simulink model "SWC_FDC_type"  (R2021b)
settings: Solver=FixedStepDiscrete  StartTime=0.0  StopTime=10.0  FixedStep=0.001  RelTol=1e-3
values from neighbouring files (symbols this model uses):
  DID_VCUKey = uint16(0x0202)    [vcu_local_hdr.m]
  DID_XWD = uint16(513)    [vcu_local_hdr.m]
  DIDLen_DKCKey = uint16(8)    [vcu_local_hdr.m]
  DIDLen_DynoMode = uint16(1)    [vcu_local_hdr.m]
  DIDLen_LFLowPresThre = uint16(1)    [vcu_local_hdr.m]
  DIDLen_LFSensorID = uint16(4)    [vcu_local_hdr.m]
  DIDLen_LRLowPresThre = uint16(1)    [vcu_local_hdr.m]
  DIDLen_LRSensorID = uint16(4)    [vcu_local_hdr.m]
  DIDLen_RFLowPresThre = uint16(1)    [vcu_local_hdr.m]
  DIDLen_RFSensorID = uint16(4)    [vcu_local_hdr.m]
  DIDLen_RRLowPresThre = uint16(1)    [vcu_local_hdr.m]
  DIDLen_RRSensorID = uint16(4)    [vcu_local_hdr.m]
  DIDLen_SensorMode = uint16(1)    [vcu_local_hdr.m]
  DIDLen_TPMSLearnSta = uint16(1)    [vcu_local_hdr.m]
  DIDLen_WhlPres = uint16(4)    [vcu_local_hdr.m]
  DIDLen_WhlSensorBattSta = uint16(1)    [vcu_local_hdr.m]
  DIDLen_WhlTmp = uint16(4)    [vcu_local_hdr.m]
  DIDLen_XWDMode = uint16(1)    [vcu_local_hdr.m]
  DIDNum_DKCKey = uint16(0x0202)    [vcu_local_hdr.m]
  DIDNum_DynoMode = uint16(0x0203)    [vcu_local_hdr.m]
  DIDNum_LFLowPresThre = uint16(0x0B08)    [vcu_local_hdr.m]
  DIDNum_LFSensorID = uint16(0x0B01)    [vcu_local_hdr.m]
  DIDNum_LRLowPresThre = uint16(0x0B0A)    [vcu_local_hdr.m]
  DIDNum_LRSensorID = uint16(0x0B03)    [vcu_local_hdr.m]
  DIDNum_RFLowPresThre = uint16(0x0B09)    [vcu_local_hdr.m]
  DIDNum_RFSensorID = uint16(0x0B02)    [vcu_local_hdr.m]
  DIDNum_RRLowPresThre = uint16(0x0B0B)    [vcu_local_hdr.m]
  DIDNum_RRSensorID = uint16(0x0B04)    [vcu_local_hdr.m]
  DIDNum_SensorMode = uint16(0x0B0C)    [vcu_local_hdr.m]
  DIDNum_TPMSLearnSta = uint16(0x0B0D)    [vcu_local_hdr.m]
  DIDNum_WhlPres = uint16(0x0B05)    [vcu_local_hdr.m]
  DIDNum_WhlSensorBattSta = uint16(0x0B07)    [vcu_local_hdr.m]
  DIDNum_WhlTmp = uint16(0x0B06)    [vcu_local_hdr.m]
  DIDNum_XWDMode = uint16(0x0201)    [vcu_local_hdr.m]
  DIDVCUKeyLength = uint16(8)    [vcu_local_hdr.m]
  ENUM_DRIVETRAIN_AWD = uint8(  2  )    [vcu_local_hdr.m]
  ENUM_DRIVETRAIN_FWD = uint8(  1  )    [vcu_local_hdr.m]
  ENUM_DRIVETRAIN_RWD = uint8(  0  )    [vcu_local_hdr.m]
  ENUM_TPMSLearnStatus_LEARNED = uint8(  1  )    [vcu_local_hdr.m]
  ENUM_TPMSLearnStatus_LEARNFAIL = uint8(  2  )    [vcu_local_hdr.m]
  ENUM_TPMSLearnStatus_NOTLEARN = uint8(  0  )    [vcu_local_hdr.m]
  ENUM_TPMSSTA_FAT = uint8(  8  )    [vcu_local_hdr.m]
  ENUM_TPMSSTA_LOWBATTERY = uint8(  2  )    [vcu_local_hdr.m]
  FALSE = boolean( 0 )    [vcu_local_hdr.m]
  ONE_INT = uint8(1)    [vcu_local_hdr.m]
  P_boolean = 0.0    [APPTypes.sldd]
  TRUE = boolean( 1 )    [vcu_local_hdr.m]
  ZERO_FLOAT = single(0)    [vcu_local_hdr.m]
  ZERO_INT = uint8(0)    [vcu_local_hdr.m]
undefined symbols (not defined in the file or in its folder): f32_ApsOutVehSpdSig, KHAL_DKCDecryptEnable_flg_ovrdflg, KHAL_DKCDecryptEnable_flg_ovrdval, KHAL_RandomNumberY1_enum, KHAL_RandomNumberY2_enum, KHAL_RandomNumberY_ovrdflg, KHAL_TPMSRESBUTT_flg_ovrdflg, KHAL_TPMSRESBUTT_flg_ovrdval, R_DIDWriteCDD_CSOP_DIDSet_DKCKey, R_DIDWriteCDD_CSOP_DIDSet_DynoMode, R_DIDWriteCDD_CSOP_DIDSet_LFLowPresThre, R_DIDWriteCDD_CSOP_DIDSet_LFSensorID, R_DIDWriteCDD_CSOP_DIDSet_LRLowPresThre, R_DIDWriteCDD_CSOP_DIDSet_LRSensorID, R_DIDWriteCDD_CSOP_DIDSet_RFLowPresThre, R_DIDWriteCDD_CSOP_DIDSet_RFSensorID, R_DIDWriteCDD_CSOP_DIDSet_RRLowPresThre, R_DIDWriteCDD_CSOP_DIDSet_RRSensorID, R_DIDWriteCDD_CSOP_DIDSet_SensorMode, R_DIDWriteCDD_CSOP_DIDSet_TPMSLearnSta, R_DIDWriteCDD_CSOP_DIDSet_WhlPres, R_DIDWriteCDD_CSOP_DIDSet_WhlSensorBattSta, R_DIDWriteCDD_CSOP_DIDSet_WhlTmp, R_DIDWriteCDD_CSOP_DIDSet_XWDMode, R_E2E_CAN3_VCU1_CSOP_Write_CAN3_VCU1, R_E2E_CAN4_VCU1_CSOP_Write_CAN4_VCU1, R_FDCCDD_Inner_CSOP_FDC_AppCallSleep, R_HALIN_IMU_CSOP_IMUSetSta, R_HALINCDD_CSOP_PAS_Handler, R_HALINCDD_CSOP_UDS_Main, R_HALOUT_APS_CSOP_ApsOutput, R_HALOUTCDD_CSOP_AppNmStateReq, R_HALOUTCDD_CSOP_IVIReset, R_HALOUTCDD_CSOP_SetAcoreRebootCmdACK, R_HALOUTCDD_CSOP_SetSysPwrStat, R_HALOUTCDD_CSOP_SleepRequest, R_NVMReadCDD_Inner_NVM_ReadOperation, R_NVMWriteCDD_Inner_NVM_WriteOperation, R_UDSCDD_CSOP_DdmRestartOperationCycle, R_WDGCDD_CSOP_Call_Watchdog, R_WDGCDD_CSOP_Call_WDG_AppEnd, R_WDGCDD_CSOP_Call_WDG_AppStart, u16_DIDLen_DKCKey, u16_DIDLen_DynoMode, u16_DIDLen_LFLowPresThre, u16_DIDLen_LFSensorID, u16_DIDLen_LRLowPresThre, u16_DIDLen_LRSensorID, u16_DIDLen_RFLowPresThre, u16_DIDLen_RFSensorID, u16_DIDLen_RRLowPresThre, u16_DIDLen_RRSensorID, u16_DIDLen_SensorMode, u16_DIDLen_TPMSLearnSta, u16_DIDLen_WhlPres, u16_DIDLen_WhlSensorBattSta, u16_DIDLen_WhlTmp, u16_DIDLen_XWDMode, u16_DIDNum_DKCKey, u16_DIDNum_DynoMode ... (+42)
libraries: simulink x215, FVT_lib x137, hcu_lib x12, hdlsllib x9, app x1, halin x1, halout x1, inp x1, outp x1
(part 1 of 11)
settings Model: DataDictionary=APPTypes.sldd  Creator=FVT23118  LastModifiedBy=FVT23118
settings DataIOCC: SaveFormat=StructureWithTime
settings OptimizationCC: DefaultParameterBehavior=Inlined  EnhancedBackFolding=on  PassReuseOutputArgsAs=Individual arguments  ZeroExternalMemoryAtStartup=off  ZeroInternalMemoryAtStartup=off  OptimizeBlockOrder=speed  DifferentSizesBufferReuse=on  OptimizationCustomize=off  EfficientTunableParamExpr=on
settings DebuggingCC: ParameterTunabilityLossMsg=error
settings HardwareCC: ProdBitPerPointer=32  ProdBitPerSizeT=32  ProdBitPerPtrDiffT=32  ProdLargestAtomicInteger=Long  ProdLargestAtomicFloat=Double  ProdWordSize=32  ProdLongLongMode=on  ProdHWDeviceType=ARM Compatible->ARM Cortex-M
settings ModelReferenceCC: ModelReferenceNumInstancesAllowed=Single
settings SFSimCC: MATLABDynamicMemAlloc=off
settings RTWCC: Description=AUTOSAR  SystemTargetFile=autosar.tlc  GenCodeOnly=on  TemplateMakefile=ert_default_tmf  PortableWordSizes=on
settings CodeAppCC: ForceParamTrailComments=on  IgnoreCustomStorageClasses=off  OperatorAnnotations=on  SimulinkDataObjDesc=on  SFDataObjDesc=on  InsertBlockDesc=on
settings STFCustomTargetCC: TargetLangStandard=C99 (ISO)  MultiwordLength=256  ParMdlRefBuildCompliant=on  CompOptLevelCompliant=on  IncludeMdlTerminateFcn=off  CombineOutputUpdateFcns=on  SuppressErrorStatus=on  ERTCustomFileBanners=on  SupportNonFinite=off  SupportComplex=off  SupportContinuousTime=off  SupportNonInlinedSFcns=off  RemoveResetFunc=on  MATLABClassNameForMDSCustomization=Simulink.SoftwareTarget.ERTCustomization  AutosarCompliant=on  GRTInterface=off  UseToolchainInfoCompliant=on  LookupTableObjectStructAxisOrder=2,1,3,4,...  LUTObjectStructOrderEvenSpacing=Size,Table,Breakpoints  SystemTargetFile=autosar.tlc
settings ERTTargetCC: TargetLangStandard=C99 (ISO)  ConcurrentExecutionCompliant=off  IncludeMdlTerminateFcn=off  SuppressErrorStatus=on  SupportNonFinite=off  SupportComplex=off  ModelStepFunctionPrototypeControlCompliant=off  CPPClassGenCompliant=off  AutosarCompliant=on  LookupTableObjectStructAxisOrder=2,1,3,4,...  LUTObjectStructOrderEvenSpacing=Size,Table,Breakpoints  GenerateASAP2=on  InlinedParameterPlacement=NonHierarchical  ERTCustomFileTemplate=example_file_process.tlc  ConvertIfToSwitch=off  SuppressUnreachableDefaultCases=off  BooleanTrueId=true_MatlabRTW  BooleanFalseId=false_MatlabRTW

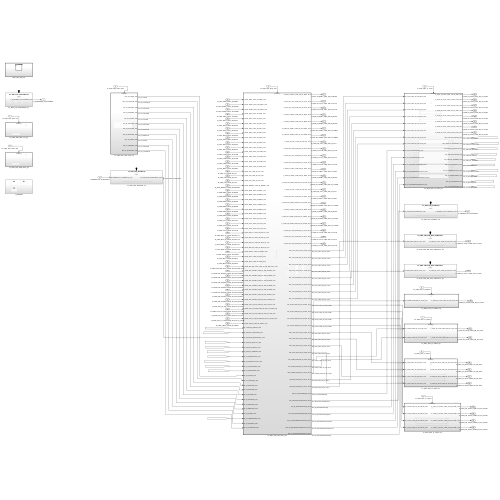
[thumbnail: Simulink's stored preview of the top-level diagram]
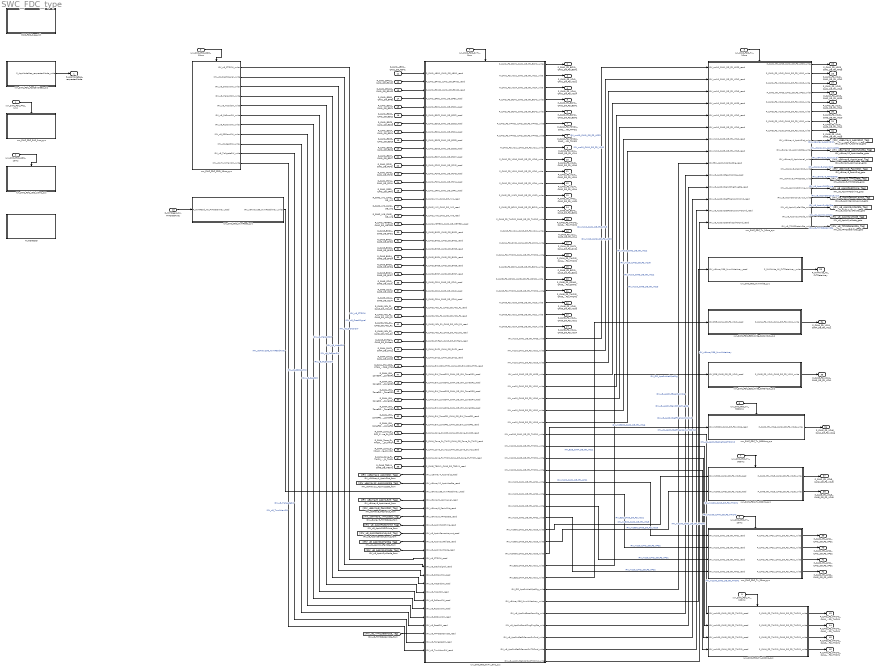
== system SWC_FDC_type ==
  run_SWC_FDC_PAS_1ms : Inport  SampleTime=0.001  OutputFunctionCall=on
  run_SWC_FDC_UDS_10ms : Inport  Port=2  SampleTime=0.01  OutputFunctionCall=on
  run_SWC_FDC_CDD_10ms : Inport  Port=3  SampleTime=0.01  OutputFunctionCall=on
  run_SWC_FDC_RxTx_5ms : Inport  Port=4  SampleTime=0.005  OutputFunctionCall=on
  run_SWC_FDC_Tx_10ms : Inport  Port=5  SampleTime=0.01  OutputFunctionCall=on
  run_SWC_FDC_Tx_5000ms : Inport  Port=6  SampleTime=5  OutputFunctionCall=on
  run_SWC_FDC_Tx_500ms : Inport  Port=7  SampleTime=0.5  OutputFunctionCall=on
  run_SWC_FDC_Tx_20ms : Inport  Port=8  SampleTime=0.02  OutputFunctionCall=on
  run_SWC_FDC_Tx_100ms : Inport  Port=9  SampleTime=0.1  OutputFunctionCall=on
  R_NVMRead_NV_FVTDataArray : Inport  Port=10  OutDataTypeStr=uint8  PortDimensions=256
  R_CAN1_ABM1_CAN1_SG_ABM1 : Inport  Port=11  OutDataTypeStr=Bus: DT_CAN1_SG_ABM1  PortDimensions=1  BusOutputAsStruct=on
  R_CAN1_EPAS1_CAN1_SG_EPAS1 : Inport  Port=12  OutDataTypeStr=Bus: DT_CAN1_SG_EPAS1  PortDimensions=1  BusOutputAsStruct=on
  R_CAN1_EPAS2_CAN1_SG_EPAS2 : Inport  Port=13  OutDataTypeStr=Bus: DT_CAN1_SG_EPAS2  PortDimensions=1  BusOutputAsStruct=on
  R_CAN1_EPB1_CAN1_SG_EPB1 : Inport  Port=14  OutDataTypeStr=Bus: DT_CAN1_SG_EPB1  PortDimensions=1  BusOutputAsStruct=on
  R_CAN1_ESC1_CAN1_SG_ESC1 : Inport  Port=15  OutDataTypeStr=Bus: DT_CAN1_SG_ESC1  PortDimensions=1  BusOutputAsStruct=on
  R_CAN1_ESC2_CAN1_SG_ESC2 : Inport  Port=16  OutDataTypeStr=Bus: DT_CAN1_SG_ESC2  PortDimensions=1  BusOutputAsStruct=on
  R_CAN1_ESC3_CAN1_SG_ESC3 : Inport  Port=17  OutDataTypeStr=Bus: DT_CAN1_SG_ESC3  PortDimensions=1  BusOutputAsStruct=on
  R_CAN1_ESC4_CAN1_SG_ESC4 : Inport  Port=18  OutDataTypeStr=Bus: DT_CAN1_SG_ESC4  PortDimensions=1  BusOutputAsStruct=on
  R_CAN1_ESC5_CAN1_SG_ESC5 : Inport  Port=19  OutDataTypeStr=Bus: DT_CAN1_SG_ESC5  PortDimensions=1  BusOutputAsStruct=on
  R_CAN1_ESC6_CAN1_SG_ESC6 : Inport  Port=20  OutDataTypeStr=Bus: DT_CAN1_SG_ESC6  PortDimensions=1  BusOutputAsStruct=on
  R_CAN1_ESC7_CAN1_SG_ESC7 : Inport  Port=21  OutDataTypeStr=Bus: DT_CAN1_SG_ESC7  PortDimensions=1  BusOutputAsStruct=on
  R_CAN1_FCM2_CAN1_SG_FCM2 : Inport  Port=22  OutDataTypeStr=Bus: DT_CAN1_SG_FCM2  PortDimensions=1  BusOutputAsStruct=on
  R_CAN1_FCM3_CAN1_SG_FCM3 : Inport  Port=23  OutDataTypeStr=Bus: DT_CAN1_SG_FCM3  PortDimensions=1  BusOutputAsStruct=on
  R_CAN1_FCM4_CAN1_SG_FCM4 : Inport  Port=24  OutDataTypeStr=Bus: DT_CAN1_SG_FCM4  PortDimensions=1  BusOutputAsStruct=on
  R_CAN1_SRR1_CAN1_SG_SRR1 : Inport  Port=25  OutDataTypeStr=Bus: DT_CAN1_SG_SRR1  PortDimensions=1  BusOutputAsStruct=on
  R_CAN2_IVI1_CAN2_SG_IVI1 : Inport  Port=26  OutDataTypeStr=Bus: DT_CAN2_SG_IVI1  PortDimensions=1  BusOutputAsStruct=on
  R_CAN2_IVI2_CAN2_SG_IVI2 : Inport  Port=27  OutDataTypeStr=Bus: DT_CAN2_SG_IVI2  PortDimensions=1  BusOutputAsStruct=on
  R_CAN2_IVI6_CAN2_SG_IVI6 : Inport  Port=28  OutDataTypeStr=Bus: DT_CAN2_SG_IVI6  PortDimensions=1  BusOutputAsStruct=on
  R_CAN2_METER1_CAN2_SG_METER1 : Inport  Port=29  OutDataTypeStr=Bus: DT_CAN2_SG_METER1  PortDimensions=1  BusOutputAsStruct=on
  R_CAN3_BMS1_CAN3_SG_BMS1 : Inport  Port=30  OutDataTypeStr=Bus: DT_CAN3_SG_BMS1  PortDimensions=1  BusOutputAsStruct=on
  R_CAN3_BMS2_CAN3_SG_BMS2 : Inport  Port=31  OutDataTypeStr=Bus: DT_CAN3_SG_BMS2  PortDimensions=1  BusOutputAsStruct=on
  R_CAN3_BMS3_CAN3_SG_BMS3 : Inport  Port=32  OutDataTypeStr=Bus: DT_CAN3_SG_BMS3  PortDimensions=1  BusOutputAsStruct=on
  R_CAN3_BMS4_CAN3_SG_BMS4 : Inport  Port=33  OutDataTypeStr=Bus: DT_CAN3_SG_BMS4  PortDimensions=1  BusOutputAsStruct=on
  R_CAN3_BMS6_CAN3_SG_BMS6 : Inport  Port=34  OutDataTypeStr=Bus: DT_CAN3_SG_BMS6  PortDimensions=1  BusOutputAsStruct=on
  R_CAN3_BMS7_CAN3_SG_BMS7 : Inport  Port=35  OutDataTypeStr=Bus: DT_CAN3_SG_BMS7  PortDimensions=1  BusOutputAsStruct=on
  R_CAN3_CCU1_CAN3_SG_CCU1 : Inport  Port=36  OutDataTypeStr=Bus: DT_CAN3_SG_CCU1  PortDimensions=1  BusOutputAsStruct=on
  R_CAN3_CCU2_CAN3_SG_CCU2 : Inport  Port=37  OutDataTypeStr=Bus: DT_CAN3_SG_CCU2  PortDimensions=1  BusOutputAsStruct=on
  R_CAN3_CCU4_CAN3_SG_CCU4 : Inport  Port=38  OutDataTypeStr=Bus: DT_CAN3_SG_CCU4  PortDimensions=1  BusOutputAsStruct=on
  R_CAN3_MCU_F1_CAN3_SG_MCU_F1 : Inport  Port=39  OutDataTypeStr=Bus: DT_CAN3_SG_MCU_F1  PortDimensions=1  BusOutputAsStruct=on
  R_CAN3_MCU_F2_CAN3_SG_MCU_F2 : Inport  Port=40  OutDataTypeStr=Bus: DT_CAN3_SG_MCU_F2  PortDimensions=1  BusOutputAsStruct=on
  R_CAN3_MCU_R1_CAN3_SG_MCU_R1 : Inport  Port=41  OutDataTypeStr=Bus: DT_CAN3_SG_MCU_R1  PortDimensions=1  BusOutputAsStruct=on
  R_CAN3_MCU_R2_CAN3_SG_MCU_R2 : Inport  Port=42  OutDataTypeStr=Bus: DT_CAN3_SG_MCU_R2  PortDimensions=1  BusOutputAsStruct=on
  R_CAN3_Shifter1_CAN3_SG_Shifter1 : Inport  Port=43  OutDataTypeStr=Bus: DT_CAN3_SG_Shifter1  PortDimensions=1  BusOutputAsStruct=on
  R_CAN4_DKC1_CAN4_SG_DKC1 : Inport  Port=44  OutDataTypeStr=Bus: DT_CAN4_SG_DKC1  PortDimensions=1  BusOutputAsStruct=on
  R_CAN4_DKC2_CAN4_SG_DKC2 : Inport  Port=45  OutDataTypeStr=Bus: DT_CAN4_SG_DKC2  PortDimensions=1  BusOutputAsStruct=on
  R_CAN4_GW_ZDR_PTG1_CAN4_SG_GW_ZDR_PTG1 : Inport  Port=46  OutDataTypeStr=Bus: DT_CAN4_SG_GW_ZDR_PTG1  PortDimensions=1  BusOutputAsStruct=on
  R_CAN4_GW_ZoneDR1_CAN4_SG_GW_ZoneDR1 : Inport  Port=47  OutDataTypeStr=Bus: DT_CAN4_SG_GW_ZoneDR1  PortDimensions=1  BusOutputAsStruct=on
  R_CAN4_GW_ZoneDR2_CAN4_SG_GW_ZoneDR2 : Inport  Port=48  OutDataTypeStr=Bus: DT_CAN4_SG_GW_ZoneDR2  PortDimensions=1  BusOutputAsStruct=on
  R_CAN4_GW_ZoneDR3_CAN4_SG_GW_ZoneDR3 : Inport  Port=49  OutDataTypeStr=Bus: DT_CAN4_SG_GW_ZoneDR3  PortDimensions=1  BusOutputAsStruct=on
  R_CAN4_GW_ZoneDR4_CAN4_SG_GW_ZoneDR4 : Inport  Port=50  OutDataTypeStr=Bus: DT_CAN4_SG_GW_ZoneDR4  PortDimensions=1  BusOutputAsStruct=on
  R_CAN4_GW_ZoneDR6_CAN4_SG_GW_ZoneDR6 : Inport  Port=51  OutDataTypeStr=Bus: DT_CAN4_SG_GW_ZoneDR6  PortDimensions=1  BusOutputAsStruct=on
  R_CAN4_GW_ZoneFR1_CAN4_SG_GW_ZoneFR1 : Inport  Port=52  OutDataTypeStr=Bus: DT_CAN4_SG_GW_ZoneFR1  PortDimensions=1  BusOutputAsStruct=on
  R_CAN4_GW_ZoneFR2_CAN4_SG_GW_ZoneFR2 : Inport  Port=53  OutDataTypeStr=Bus: DT_CAN4_SG_GW_ZoneFR2  PortDimensions=1  BusOutputAsStruct=on
  R_CAN4_Zone_Dr_SCP_CAN4_SG_Zone_Dr_SCP : Inport  Port=54  OutDataTypeStr=Bus: DT_CAN4_SG_Zone_Dr_SCP  PortDimensions=1  BusOutputAsStruct=on
  R_CAN4_Zone_Dr_THCM_CAN4_SG_Zone_Dr_THCM : Inport  Port=55  OutDataTypeStr=Bus: DT_CAN4_SG_Zone_Dr_THCM  PortDimensions=1  BusOutputAsStruct=on
  R_CAN4_Zone_Dr_VCU_CAN4_SG_Zone_Dr_VCU : Inport  Port=56  OutDataTypeStr=Bus: DT_CAN4_SG_Zone_Dr_VCU  PortDimensions=1  BusOutputAsStruct=on
  R_CAN4_Zone_Fr_THCM_CAN4_SG_Zone_Fr_THCM : Inport  Port=57  OutDataTypeStr=Bus: DT_CAN4_SG_Zone_Fr_THCM  PortDimensions=1  BusOutputAsStruct=on
  R_CAN5_TBOX1_CAN5_SG_TBOX1 : Inport  Port=58  OutDataTypeStr=Bus: DT_CAN5_SG_TBOX1  PortDimensions=1  BusOutputAsStruct=on
  P_WDGCDD : Subsystem
  SWC_FDC_type_Init : Subsystem
  run_SWC_FDC_AppCallSleep_sys : Subsystem
  run_SWC_FDC_CDD_10ms_sys : Subsystem
  run_SWC_FDC_E2E_Write_CAN3VCU1_sys : Subsystem
  run_SWC_FDC_E2E_Write_CAN4VCU1_sys : Subsystem
  run_SWC_FDC_NvmRead_sys : Subsystem
  run_SWC_FDC_NvmWrite_sys : Subsystem
  run_SWC_FDC_PAS_1ms_sys : Subsystem
  run_SWC_FDC_RxTx_5ms_sys : Subsystem
  run_SWC_FDC_Tx_100ms_sys : Subsystem
  run_SWC_FDC_Tx_10ms_sys : Subsystem
  run_SWC_FDC_Tx_20ms_sys : Subsystem
  run_SWC_FDC_Tx_5000ms_sys : Subsystem
  run_SWC_FDC_Tx_500ms_sys : Subsystem
  run_SWC_FDC_UDS_10ms_sys : Subsystem
  P_AppModeReq_requestedMode : Outport  OutDataTypeStr=Enum: AppModeRequestType  PortDimensions=1
  P_CAN1_FD_BCM1_CAN1_SG_FD_BCM1 : Outport  Port=2  OutDataTypeStr=Bus: DT_CAN1_SG_FD_BCM1  PortDimensions=1  BusOutputAsStruct=on
  P_CAN1_FD_VCU1_CAN1_SG_FD_VCU1 : Outport  Port=3  OutDataTypeStr=Bus: DT_CAN1_SG_FD_VCU1  PortDimensions=1  BusOutputAsStruct=on
  P_CAN1_FD_VCU4_CAN1_SG_FD_VCU4 : Outport  Port=4  OutDataTypeStr=Bus: DT_CAN1_SG_FD_VCU4  PortDimensions=1  BusOutputAsStruct=on
  P_CAN2_FD_BCM1_CAN2_SG_FD_BCM1 : Outport  Port=5  OutDataTypeStr=Bus: DT_CAN2_SG_FD_BCM1  PortDimensions=1  BusOutputAsStruct=on
  P_CAN2_FD_BCM2_CAN2_SG_FD_BCM2 : Outport  Port=6  OutDataTypeStr=Bus: DT_CAN2_SG_FD_BCM2  PortDimensions=1  BusOutputAsStruct=on
  P_CAN2_FD_TPMS1_CAN2_SG_FD_TPMS1 : Outport  Port=7  OutDataTypeStr=Bus: DT_CAN2_SG_FD_TPMS1  PortDimensions=1  BusOutputAsStruct=on
  P_CAN2_FD_TPMS2_CAN2_SG_FD_TPMS2 : Outport  Port=8  OutDataTypeStr=Bus: DT_CAN2_SG_FD_TPMS2  PortDimensions=1  BusOutputAsStruct=on
  P_CAN2_FD_V2L1_CAN2_SG_FD_V2L1 : Outport  Port=9  OutDataTypeStr=Bus: DT_CAN2_SG_FD_V2L1  PortDimensions=1  BusOutputAsStruct=on
  P_CAN2_FD_VCU0_CAN2_SG_FD_VCU0 : Outport  Port=10  OutDataTypeStr=Bus: DT_CAN2_SG_FD_VCU0  PortDimensions=1  BusOutputAsStruct=on
  P_CAN2_FD_VCU1_CAN2_SG_FD_VCU1 : Outport  Port=11  OutDataTypeStr=Bus: DT_CAN2_SG_FD_VCU1  PortDimensions=1  BusOutputAsStruct=on
  P_CAN2_FD_VCU4_CAN2_SG_FD_VCU4 : Outport  Port=12  OutDataTypeStr=Bus: DT_CAN2_SG_FD_VCU4  PortDimensions=1  BusOutputAsStruct=on
  P_CAN2_FD_VMC1_CAN2_SG_FD_VMC1 : Outport  Port=13  OutDataTypeStr=Bus: DT_CAN2_SG_FD_VMC1  PortDimensions=1  BusOutputAsStruct=on
  P_CAN3_FD_BCM1_CAN3_SG_FD_BCM1 : Outport  Port=14  OutDataTypeStr=Bus: DT_CAN3_SG_FD_BCM1  PortDimensions=1  BusOutputAsStruct=on
  P_CAN3_FD_THCM2_CAN3_SG_FD_THCM2 : Outport  Port=15  OutDataTypeStr=Bus: DT_CAN3_SG_FD_THCM2  PortDimensions=1  BusOutputAsStruct=on
  P_CAN3_FD_V2L1_CAN3_SG_FD_V2L1 : Outport  Port=16  OutDataTypeStr=Bus: DT_CAN3_SG_FD_V2L1  PortDimensions=1  BusOutputAsStruct=on
  P_CAN4_FD_DKC1_CAN4_SG_FD_DKC1 : Outport  Port=17  OutDataTypeStr=Bus: DT_CAN4_SG_FD_DKC1  PortDimensions=1  BusOutputAsStruct=on
  P_CAN4_FD_THCM2_CAN4_SG_FD_THCM2 : Outport  Port=18  OutDataTypeStr=Bus: DT_CAN4_SG_FD_THCM2  PortDimensions=1  BusOutputAsStruct=on
  P_CAN5_FD_BCM1_CAN5_SG_FD_BCM1 : Outport  Port=19  OutDataTypeStr=Bus: DT_CAN5_SG_FD_BCM1  PortDimensions=1  BusOutputAsStruct=on
  P_CAN5_FD_CONN1_CAN5_SG_FD_CONN1 : Outport  Port=20  OutDataTypeStr=Bus: DT_CAN5_SG_FD_CONN1  PortDimensions=1  BusOutputAsStruct=on
  P_CAN5_FD_THCM2_CAN5_SG_FD_THCM2 : Outport  Port=21  OutDataTypeStr=Bus: DT_CAN5_SG_FD_THCM2  PortDimensions=1  BusOutputAsStruct=on
  P_CAN5_FD_VCU0_CAN5_SG_FD_VCU0 : Outport  Port=22  OutDataTypeStr=Bus: DT_CAN5_SG_FD_VCU0  PortDimensions=1  BusOutputAsStruct=on
  P_CAN5_FD_VCU1_CAN5_SG_FD_VCU1 : Outport  Port=23  OutDataTypeStr=Bus: DT_CAN5_SG_FD_VCU1  PortDimensions=1  BusOutputAsStruct=on
  P_CAN5_FD_VCU4_CAN5_SG_FD_VCU4 : Outport  Port=24  OutDataTypeStr=Bus: DT_CAN5_SG_FD_VCU4  PortDimensions=1  BusOutputAsStruct=on
  P_CAN1_FD_APS3_CAN1_SG_FD_APS3 : Outport  Port=25  OutDataTypeStr=Bus: DT_CAN1_SG_FD_APS3  PortDimensions=1  BusOutputAsStruct=on
  P_CAN1_FD_VCU2_CAN1_SG_FD_VCU2 : Outport  Port=26  OutDataTypeStr=Bus: DT_CAN1_SG_FD_VCU2  PortDimensions=1  BusOutputAsStruct=on
  P_CAN1_FD_VCU3_CAN1_SG_FD_VCU3 : Outport  Port=27  OutDataTypeStr=Bus: DT_CAN1_SG_FD_VCU3  PortDimensions=1  BusOutputAsStruct=on
  P_CAN2_FD_APS3_CAN2_SG_FD_APS3 : Outport  Port=28  OutDataTypeStr=Bus: DT_CAN2_SG_FD_APS3  PortDimensions=1  BusOutputAsStruct=on
  P_CAN2_FD_VCU2_CAN2_SG_FD_VCU2 : Outport  Port=29  OutDataTypeStr=Bus: DT_CAN2_SG_FD_VCU2  PortDimensions=1  BusOutputAsStruct=on
  P_CAN3_FD_VCU0_CAN3_SG_FD_VCU0 : Outport  Port=30  OutDataTypeStr=Bus: DT_CAN3_SG_FD_VCU0  PortDimensions=1  BusOutputAsStruct=on
  P_CAN3_FD_VCU2_CAN3_SG_FD_VCU2 : Outport  Port=31  OutDataTypeStr=Bus: DT_CAN3_SG_FD_VCU2  PortDimensions=1  BusOutputAsStruct=on
  P_CAN5_FD_VCU3_CAN5_SG_FD_VCU3 : Outport  Port=32  OutDataTypeStr=Bus: DT_CAN5_SG_FD_VCU3  PortDimensions=1  BusOutputAsStruct=on
  P_NVMWrite_NV_FVTDataArray : Outport  Port=33  OutDataTypeStr=uint8  PortDimensions=256
  P_CAN4_FD_VCU1_CAN4_SG_FD_VCU1 : Outport  Port=34  OutDataTypeStr=Bus: DT_CAN4_SG_FD_VCU1  PortDimensions=1  BusOutputAsStruct=on
  P_CAN3_FD_VCU1_CAN3_SG_FD_VCU1 : Outport  Port=35  OutDataTypeStr=Bus: DT_CAN3_SG_FD_VCU1  PortDimensions=1  BusOutputAsStruct=on
  P_CAN2_FD_VCU6_CAN2_SG_FD_VCU6 : Outport  Port=36  OutDataTypeStr=Bus: DT_CAN2_SG_FD_VCU6  PortDimensions=1  BusOutputAsStruct=on
  P_CAN2_FD_VCU5_CAN2_SG_FD_VCU5 : Outport  Port=37  OutDataTypeStr=Bus: DT_CAN2_SG_FD_VCU5  PortDimensions=1  BusOutputAsStruct=on
  P_CAN5_FD_VCU5_CAN5_SG_FD_VCU5 : Outport  Port=38  OutDataTypeStr=Bus: DT_CAN5_SG_FD_VCU5  PortDimensions=1  BusOutputAsStruct=on
  P_CAN1_FD_APS1_CAN1_SG_FD_APS1 : Outport  Port=39  OutDataTypeStr=Bus: DT_CAN1_SG_FD_APS1  PortDimensions=1  BusOutputAsStruct=on
  P_CAN1_FD_APS2_CAN1_SG_FD_APS2 : Outport  Port=40  OutDataTypeStr=Bus: DT_CAN1_SG_FD_APS2  PortDimensions=1  BusOutputAsStruct=on
  P_CAN2_FD_APS1_CAN2_SG_FD_APS1 : Outport  Port=41  OutDataTypeStr=Bus: DT_CAN2_SG_FD_APS1  PortDimensions=1  BusOutputAsStruct=on
  P_CAN2_FD_APS2_CAN2_SG_FD_APS2 : Outport  Port=42  OutDataTypeStr=Bus: DT_CAN2_SG_FD_APS2  PortDimensions=1  BusOutputAsStruct=on
  P_CAN1_FD_THCM1_CAN1_SG_FD_THCM1 : Outport  Port=43  OutDataTypeStr=Bus: DT_CAN1_SG_FD_THCM1  PortDimensions=1  BusOutputAsStruct=on
  P_CAN2_FD_THCM1_CAN2_SG_FD_THCM1 : Outport  Port=44  OutDataTypeStr=Bus: DT_CAN2_SG_FD_THCM1  PortDimensions=1  BusOutputAsStruct=on
  P_CAN3_FD_THCM1_CAN3_SG_FD_THCM1 : Outport  Port=45  OutDataTypeStr=Bus: DT_CAN3_SG_FD_THCM1  PortDimensions=1  BusOutputAsStruct=on
  P_CAN4_FD_THCM1_CAN4_SG_FD_THCM1 : Outport  Port=46  OutDataTypeStr=Bus: DT_CAN4_SG_FD_THCM1  PortDimensions=1  BusOutputAsStruct=on
  wires:
  run_SWC_FDC_AppCallSleep_sys/1(P_AppModeReq_requestedMode_write) -> P_AppModeReq_requestedMode/1
  R_NVMRead_NV_FVTDataArray/1 -> run_SWC_FDC_NvmRead_sys/1(R_NVMRead_NV_FVTDataArray_read)
  R_CAN1_ABM1_CAN1_SG_ABM1/1 -> run_SWC_FDC_RxTx_5ms_sys/1(R_CAN1_ABM1_CAN1_SG_ABM1_read)
  R_CAN1_EPAS1_CAN1_SG_EPAS1/1 -> run_SWC_FDC_RxTx_5ms_sys/2(R_CAN1_EPAS1_CAN1_SG_EPAS1_read)
  R_CAN1_EPAS2_CAN1_SG_EPAS2/1 -> run_SWC_FDC_RxTx_5ms_sys/3(R_CAN1_EPAS2_CAN1_SG_EPAS2_read)
  R_CAN1_EPB1_CAN1_SG_EPB1/1 -> run_SWC_FDC_RxTx_5ms_sys/4(R_CAN1_EPB1_CAN1_SG_EPB1_read)
  R_CAN1_ESC1_CAN1_SG_ESC1/1 -> run_SWC_FDC_RxTx_5ms_sys/5(R_CAN1_ESC1_CAN1_SG_ESC1_read)
  R_CAN1_ESC2_CAN1_SG_ESC2/1 -> run_SWC_FDC_RxTx_5ms_sys/6(R_CAN1_ESC2_CAN1_SG_ESC2_read)
  R_CAN1_ESC3_CAN1_SG_ESC3/1 -> run_SWC_FDC_RxTx_5ms_sys/7(R_CAN1_ESC3_CAN1_SG_ESC3_read)
  R_CAN1_ESC4_CAN1_SG_ESC4/1 -> run_SWC_FDC_RxTx_5ms_sys/8(R_CAN1_ESC4_CAN1_SG_ESC4_read)
  R_CAN1_ESC5_CAN1_SG_ESC5/1 -> run_SWC_FDC_RxTx_5ms_sys/9(R_CAN1_ESC5_CAN1_SG_ESC5_read)
  R_CAN1_ESC6_CAN1_SG_ESC6/1 -> run_SWC_FDC_RxTx_5ms_sys/10(R_CAN1_ESC6_CAN1_SG_ESC6_read)
  R_CAN1_ESC7_CAN1_SG_ESC7/1 -> run_SWC_FDC_RxTx_5ms_sys/11(R_CAN1_ESC7_CAN1_SG_ESC7_read)
  R_CAN1_FCM2_CAN1_SG_FCM2/1 -> run_SWC_FDC_RxTx_5ms_sys/12(R_CAN1_FCM2_CAN1_SG_FCM2_read)
  R_CAN1_FCM3_CAN1_SG_FCM3/1 -> run_SWC_FDC_RxTx_5ms_sys/13(R_CAN1_FCM3_CAN1_SG_FCM3_read)
  R_CAN1_FCM4_CAN1_SG_FCM4/1 -> run_SWC_FDC_RxTx_5ms_sys/14(R_CAN1_FCM4_CAN1_SG_FCM4_read)
  R_CAN1_SRR1_CAN1_SG_SRR1/1 -> run_SWC_FDC_RxTx_5ms_sys/15(R_CAN1_SRR1_CAN1_SG_SRR1_read)
  R_CAN2_IVI1_CAN2_SG_IVI1/1 -> run_SWC_FDC_RxTx_5ms_sys/16(R_CAN2_IVI1_CAN2_SG_IVI1_read)
  R_CAN2_IVI2_CAN2_SG_IVI2/1 -> run_SWC_FDC_RxTx_5ms_sys/17(R_CAN2_IVI2_CAN2_SG_IVI2_read)
  R_CAN2_IVI6_CAN2_SG_IVI6/1 -> run_SWC_FDC_RxTx_5ms_sys/18(R_CAN2_IVI6_CAN2_SG_IVI6_read)
  R_CAN2_METER1_CAN2_SG_METER1/1 -> run_SWC_FDC_RxTx_5ms_sys/19(R_CAN2_METER1_CAN2_SG_METER1_read)
  R_CAN3_BMS1_CAN3_SG_BMS1/1 -> run_SWC_FDC_RxTx_5ms_sys/20(R_CAN3_BMS1_CAN3_SG_BMS1_read)
  R_CAN3_BMS2_CAN3_SG_BMS2/1 -> run_SWC_FDC_RxTx_5ms_sys/21(R_CAN3_BMS2_CAN3_SG_BMS2_read)
  R_CAN3_BMS3_CAN3_SG_BMS3/1 -> run_SWC_FDC_RxTx_5ms_sys/22(R_CAN3_BMS3_CAN3_SG_BMS3_read)
  R_CAN3_BMS4_CAN3_SG_BMS4/1 -> run_SWC_FDC_RxTx_5ms_sys/23(R_CAN3_BMS4_CAN3_SG_BMS4_read)
  R_CAN3_BMS6_CAN3_SG_BMS6/1 -> run_SWC_FDC_RxTx_5ms_sys/24(R_CAN3_BMS6_CAN3_SG_BMS6_read)
  R_CAN3_BMS7_CAN3_SG_BMS7/1 -> run_SWC_FDC_RxTx_5ms_sys/25(R_CAN3_BMS7_CAN3_SG_BMS7_read)
  R_CAN3_CCU1_CAN3_SG_CCU1/1 -> run_SWC_FDC_RxTx_5ms_sys/26(R_CAN3_CCU1_CAN3_SG_CCU1_read)
  R_CAN3_CCU2_CAN3_SG_CCU2/1 -> run_SWC_FDC_RxTx_5ms_sys/27(R_CAN3_CCU2_CAN3_SG_CCU2_read)
  R_CAN3_CCU4_CAN3_SG_CCU4/1 -> run_SWC_FDC_RxTx_5ms_sys/28(R_CAN3_CCU4_CAN3_SG_CCU4_read)
  R_CAN3_MCU_F1_CAN3_SG_MCU_F1/1 -> run_SWC_FDC_RxTx_5ms_sys/29(R_CAN3_MCU_F1_CAN3_SG_MCU_F1_read)
  R_CAN3_MCU_F2_CAN3_SG_MCU_F2/1 -> run_SWC_FDC_RxTx_5ms_sys/30(R_CAN3_MCU_F2_CAN3_SG_MCU_F2_read)
  R_CAN3_MCU_R1_CAN3_SG_MCU_R1/1 -> run_SWC_FDC_RxTx_5ms_sys/31(R_CAN3_MCU_R1_CAN3_SG_MCU_R1_read)
  R_CAN3_MCU_R2_CAN3_SG_MCU_R2/1 -> run_SWC_FDC_RxTx_5ms_sys/32(R_CAN3_MCU_R2_CAN3_SG_MCU_R2_read)
  R_CAN3_Shifter1_CAN3_SG_Shifter1/1 -> run_SWC_FDC_RxTx_5ms_sys/33(R_CAN3_Shifter1_CAN3_SG_Shifter1_read)
  R_CAN4_DKC1_CAN4_SG_DKC1/1 -> run_SWC_FDC_RxTx_5ms_sys/34(R_CAN4_DKC1_CAN4_SG_DKC1_read)
  R_CAN4_DKC2_CAN4_SG_DKC2/1 -> run_SWC_FDC_RxTx_5ms_sys/35(R_CAN4_DKC2_CAN4_SG_DKC2_read)
  R_CAN4_GW_ZDR_PTG1_CAN4_SG_GW_ZDR_PTG1/1 -> run_SWC_FDC_RxTx_5ms_sys/36(R_CAN4_GW_ZDR_PTG1_CAN4_SG_GW_ZDR_PTG1_read)
  R_CAN4_GW_ZoneDR1_CAN4_SG_GW_ZoneDR1/1 -> run_SWC_FDC_RxTx_5ms_sys/37(R_CAN4_GW_ZoneDR1_CAN4_SG_GW_ZoneDR1_read)
  R_CAN4_GW_ZoneDR2_CAN4_SG_GW_ZoneDR2/1 -> run_SWC_FDC_RxTx_5ms_sys/38(R_CAN4_GW_ZoneDR2_CAN4_SG_GW_ZoneDR2_read)
  R_CAN4_GW_ZoneDR3_CAN4_SG_GW_ZoneDR3/1 -> run_SWC_FDC_RxTx_5ms_sys/39(R_CAN4_GW_ZoneDR3_CAN4_SG_GW_ZoneDR3_read)
  R_CAN4_GW_ZoneDR4_CAN4_SG_GW_ZoneDR4/1 -> run_SWC_FDC_RxTx_5ms_sys/40(R_CAN4_GW_ZoneDR4_CAN4_SG_GW_ZoneDR4_read)
  R_CAN4_GW_ZoneDR6_CAN4_SG_GW_ZoneDR6/1 -> run_SWC_FDC_RxTx_5ms_sys/41(R_CAN4_GW_ZoneDR6_CAN4_SG_GW_ZoneDR6_read)
  R_CAN4_GW_ZoneFR1_CAN4_SG_GW_ZoneFR1/1 -> run_SWC_FDC_RxTx_5ms_sys/42(R_CAN4_GW_ZoneFR1_CAN4_SG_GW_ZoneFR1_read)
  R_CAN4_GW_ZoneFR2_CAN4_SG_GW_ZoneFR2/1 -> run_SWC_FDC_RxTx_5ms_sys/43(R_CAN4_GW_ZoneFR2_CAN4_SG_GW_ZoneFR2_read)
  R_CAN4_Zone_Dr_SCP_CAN4_SG_Zone_Dr_SCP/1 -> run_SWC_FDC_RxTx_5ms_sys/44(R_CAN4_Zone_Dr_SCP_CAN4_SG_Zone_Dr_SCP_read)
  R_CAN4_Zone_Dr_THCM_CAN4_SG_Zone_Dr_THCM/1 -> run_SWC_FDC_RxTx_5ms_sys/45(R_CAN4_Zone_Dr_THCM_CAN4_SG_Zone_Dr_THCM_read)
  R_CAN4_Zone_Dr_VCU_CAN4_SG_Zone_Dr_VCU/1 -> run_SWC_FDC_RxTx_5ms_sys/46(R_CAN4_Zone_Dr_VCU_CAN4_SG_Zone_Dr_VCU_read)
  R_CAN4_Zone_Fr_THCM_CAN4_SG_Zone_Fr_THCM/1 -> run_SWC_FDC_RxTx_5ms_sys/47(R_CAN4_Zone_Fr_THCM_CAN4_SG_Zone_Fr_THCM_read)
  R_CAN5_TBOX1_CAN5_SG_TBOX1/1 -> run_SWC_FDC_RxTx_5ms_sys/48(R_CAN5_TBOX1_CAN5_SG_TBOX1_read)
  run_SWC_FDC_RxTx_5ms_sys/1(P_CAN1_FD_BCM1_CAN1_SG_FD_BCM1_write) -> P_CAN1_FD_BCM1_CAN1_SG_FD_BCM1/1
  run_SWC_FDC_RxTx_5ms_sys/2(P_CAN1_FD_VCU1_CAN1_SG_FD_VCU1_write) -> P_CAN1_FD_VCU1_CAN1_SG_FD_VCU1/1
  run_SWC_FDC_RxTx_5ms_sys/3(P_CAN1_FD_VCU4_CAN1_SG_FD_VCU4_write) -> P_CAN1_FD_VCU4_CAN1_SG_FD_VCU4/1
  run_SWC_FDC_RxTx_5ms_sys/4(P_CAN2_FD_BCM1_CAN2_SG_FD_BCM1_write) -> P_CAN2_FD_BCM1_CAN2_SG_FD_BCM1/1
  run_SWC_FDC_RxTx_5ms_sys/5(P_CAN2_FD_BCM2_CAN2_SG_FD_BCM2_write) -> P_CAN2_FD_BCM2_CAN2_SG_FD_BCM2/1
  run_SWC_FDC_RxTx_5ms_sys/6(P_CAN2_FD_TPMS1_CAN2_SG_FD_TPMS1_write) -> P_CAN2_FD_TPMS1_CAN2_SG_FD_TPMS1/1
  run_SWC_FDC_RxTx_5ms_sys/7(P_CAN2_FD_TPMS2_CAN2_SG_FD_TPMS2_write) -> P_CAN2_FD_TPMS2_CAN2_SG_FD_TPMS2/1
  run_SWC_FDC_RxTx_5ms_sys/8(P_CAN2_FD_V2L1_CAN2_SG_FD_V2L1_write) -> P_CAN2_FD_V2L1_CAN2_SG_FD_V2L1/1
  run_SWC_FDC_RxTx_5ms_sys/9(P_CAN2_FD_VCU0_CAN2_SG_FD_VCU0_write) -> P_CAN2_FD_VCU0_CAN2_SG_FD_VCU0/1
  run_SWC_FDC_RxTx_5ms_sys/10(P_CAN2_FD_VCU1_CAN2_SG_FD_VCU1_write) -> P_CAN2_FD_VCU1_CAN2_SG_FD_VCU1/1
  run_SWC_FDC_RxTx_5ms_sys/11(P_CAN2_FD_VCU4_CAN2_SG_FD_VCU4_write) -> P_CAN2_FD_VCU4_CAN2_SG_FD_VCU4/1
  run_SWC_FDC_RxTx_5ms_sys/12(P_CAN2_FD_VMC1_CAN2_SG_FD_VMC1_write) -> P_CAN2_FD_VMC1_CAN2_SG_FD_VMC1/1
  run_SWC_FDC_RxTx_5ms_sys/13(P_CAN3_FD_BCM1_CAN3_SG_FD_BCM1_write) -> P_CAN3_FD_BCM1_CAN3_SG_FD_BCM1/1
  run_SWC_FDC_RxTx_5ms_sys/14(P_CAN3_FD_THCM2_CAN3_SG_FD_THCM2_write) -> P_CAN3_FD_THCM2_CAN3_SG_FD_THCM2/1
  run_SWC_FDC_RxTx_5ms_sys/15(P_CAN3_FD_V2L1_CAN3_SG_FD_V2L1_write) -> P_CAN3_FD_V2L1_CAN3_SG_FD_V2L1/1
  run_SWC_FDC_RxTx_5ms_sys/16(P_CAN4_FD_DKC1_CAN4_SG_FD_DKC1_write) -> P_CAN4_FD_DKC1_CAN4_SG_FD_DKC1/1
  run_SWC_FDC_RxTx_5ms_sys/17(P_CAN4_FD_THCM2_CAN4_SG_FD_THCM2_write) -> P_CAN4_FD_THCM2_CAN4_SG_FD_THCM2/1
  run_SWC_FDC_RxTx_5ms_sys/18(P_CAN5_FD_BCM1_CAN5_SG_FD_BCM1_write) -> P_CAN5_FD_BCM1_CAN5_SG_FD_BCM1/1
  run_SWC_FDC_RxTx_5ms_sys/19(P_CAN5_FD_CONN1_CAN5_SG_FD_CONN1_write) -> P_CAN5_FD_CONN1_CAN5_SG_FD_CONN1/1
  run_SWC_FDC_RxTx_5ms_sys/20(P_CAN5_FD_THCM2_CAN5_SG_FD_THCM2_write) -> P_CAN5_FD_THCM2_CAN5_SG_FD_THCM2/1
  run_SWC_FDC_RxTx_5ms_sys/21(P_CAN5_FD_VCU0_CAN5_SG_FD_VCU0_write) -> P_CAN5_FD_VCU0_CAN5_SG_FD_VCU0/1
  run_SWC_FDC_RxTx_5ms_sys/22(P_CAN5_FD_VCU1_CAN5_SG_FD_VCU1_write) -> P_CAN5_FD_VCU1_CAN5_SG_FD_VCU1/1
  run_SWC_FDC_RxTx_5ms_sys/23(P_CAN5_FD_VCU4_CAN5_SG_FD_VCU4_write) -> P_CAN5_FD_VCU4_CAN5_SG_FD_VCU4/1
  run_SWC_FDC_Tx_10ms_sys/1(P_CAN1_FD_APS3_CAN1_SG_FD_APS3_write) -> P_CAN1_FD_APS3_CAN1_SG_FD_APS3/1
  run_SWC_FDC_Tx_10ms_sys/2(P_CAN1_FD_VCU2_CAN1_SG_FD_VCU2_write) -> P_CAN1_FD_VCU2_CAN1_SG_FD_VCU2/1
  run_SWC_FDC_Tx_10ms_sys/3(P_CAN1_FD_VCU3_CAN1_SG_FD_VCU3_write) -> P_CAN1_FD_VCU3_CAN1_SG_FD_VCU3/1
  run_SWC_FDC_Tx_10ms_sys/4(P_CAN2_FD_APS3_CAN2_SG_FD_APS3_write) -> P_CAN2_FD_APS3_CAN2_SG_FD_APS3/1
  run_SWC_FDC_Tx_10ms_sys/5(P_CAN2_FD_VCU2_CAN2_SG_FD_VCU2_write) -> P_CAN2_FD_VCU2_CAN2_SG_FD_VCU2/1
  run_SWC_FDC_Tx_10ms_sys/6(P_CAN3_FD_VCU0_CAN3_SG_FD_VCU0_write) -> P_CAN3_FD_VCU0_CAN3_SG_FD_VCU0/1
  run_SWC_FDC_Tx_10ms_sys/7(P_CAN3_FD_VCU2_CAN3_SG_FD_VCU2_write) -> P_CAN3_FD_VCU2_CAN3_SG_FD_VCU2/1
  run_SWC_FDC_Tx_10ms_sys/8(P_CAN5_FD_VCU3_CAN5_SG_FD_VCU3_write) -> P_CAN5_FD_VCU3_CAN5_SG_FD_VCU3/1
  run_SWC_FDC_NvmWrite_sys/1(P_NVMWrite_NV_FVTDataArray_write) -> P_NVMWrite_NV_FVTDataArray/1
  run_SWC_FDC_E2E_Write_CAN4VCU1_sys/1(P_CAN4_FD_VCU1_CAN4_SG_FD_VCU1_write) -> P_CAN4_FD_VCU1_CAN4_SG_FD_VCU1/1
  run_SWC_FDC_E2E_Write_CAN3VCU1_sys/1(P_CAN3_FD_VCU1_CAN3_SG_FD_VCU1_write) -> P_CAN3_FD_VCU1_CAN3_SG_FD_VCU1/1
  run_SWC_FDC_Tx_5000ms_sys/1(P_CAN2_FD_VCU6_CAN2_SG_FD_VCU6_write) -> P_CAN2_FD_VCU6_CAN2_SG_FD_VCU6/1
  run_SWC_FDC_Tx_500ms_sys/1(P_CAN2_FD_VCU5_CAN2_SG_FD_VCU5_write) -> P_CAN2_FD_VCU5_CAN2_SG_FD_VCU5/1
  run_SWC_FDC_Tx_500ms_sys/2(P_CAN5_FD_VCU5_CAN5_SG_FD_VCU5_write) -> P_CAN5_FD_VCU5_CAN5_SG_FD_VCU5/1
  run_SWC_FDC_Tx_20ms_sys/1(P_CAN1_FD_APS1_CAN1_SG_FD_APS1_write) -> P_CAN1_FD_APS1_CAN1_SG_FD_APS1/1
  run_SWC_FDC_Tx_20ms_sys/2(P_CAN1_FD_APS2_CAN1_SG_FD_APS2_write) -> P_CAN1_FD_APS2_CAN1_SG_FD_APS2/1
  run_SWC_FDC_Tx_20ms_sys/3(P_CAN2_FD_APS1_CAN2_SG_FD_APS1_write) -> P_CAN2_FD_APS1_CAN2_SG_FD_APS1/1
  run_SWC_FDC_Tx_20ms_sys/4(P_CAN2_FD_APS2_CAN2_SG_FD_APS2_write) -> P_CAN2_FD_APS2_CAN2_SG_FD_APS2/1
  run_SWC_FDC_Tx_100ms_sys/1(P_CAN1_FD_THCM1_CAN1_SG_FD_THCM1_write) -> P_CAN1_FD_THCM1_CAN1_SG_FD_THCM1/1
  run_SWC_FDC_Tx_100ms_sys/2(P_CAN2_FD_THCM1_CAN2_SG_FD_THCM1_write) -> P_CAN2_FD_THCM1_CAN2_SG_FD_THCM1/1
  run_SWC_FDC_Tx_100ms_sys/3(P_CAN3_FD_THCM1_CAN3_SG_FD_THCM1_write) -> P_CAN3_FD_THCM1_CAN3_SG_FD_THCM1/1
  run_SWC_FDC_Tx_100ms_sys/4(P_CAN4_FD_THCM1_CAN4_SG_FD_THCM1_write) -> P_CAN4_FD_THCM1_CAN4_SG_FD_THCM1/1
  run_SWC_FDC_CDD_10ms_sys/1(IRV_u8_CTDSW_write) -> run_SWC_FDC_RxTx_5ms_sys/59(IRV_u8_CTDSW_read)  "IRV_u8_CTDSW"
  run_SWC_FDC_CDD_10ms_sys/2(IRV_u8_CrashSignal_write) -> run_SWC_FDC_RxTx_5ms_sys/60(IRV_u8_CrashSignal_read)  "IRV_u8_CrashSignal"
  run_SWC_FDC_CDD_10ms_sys/3(IRV_u8_DrDoorSW_write) -> run_SWC_FDC_RxTx_5ms_sys/61(IRV_u8_DrDoorSW_read)  "IRV_u8_DrDoorSW"
  run_SWC_FDC_CDD_10ms_sys/4(IRV_u8_HazardSW_write) -> run_SWC_FDC_RxTx_5ms_sys/62(IRV_u8_HazardSW_read)  "IRV_u8_HazardSW"
  run_SWC_FDC_CDD_10ms_sys/5(IRV_u8_HoodSW_write) -> run_SWC_FDC_RxTx_5ms_sys/63(IRV_u8_HoodSW_read)  "IRV_u8_HoodSW"
  run_SWC_FDC_CDD_10ms_sys/6(IRV_u8_PsDoorSW_write) -> run_SWC_FDC_RxTx_5ms_sys/64(IRV_u8_PsDoorSW_read)  "IRV_u8_PsDoorSW"
  run_SWC_FDC_CDD_10ms_sys/7(IRV_u8_RLDoorSW_write) -> run_SWC_FDC_RxTx_5ms_sys/65(IRV_u8_RLDoorSW_read)  "IRV_u8_RLDoorSW"
  run_SWC_FDC_CDD_10ms_sys/8(IRV_u8_RRDoorSW_write) -> run_SWC_FDC_RxTx_5ms_sys/66(IRV_u8_RRDoorSW_read)  "IRV_u8_RRDoorSW"
  run_SWC_FDC_CDD_10ms_sys/9(IRV_u8_SeatSW_write) -> run_SWC_FDC_RxTx_5ms_sys/67(IRV_u8_SeatSW_read)  "IRV_u8_SeatSW"
  run_SWC_FDC_CDD_10ms_sys/10(IRV_u8_TailgateSW_write) -> run_SWC_FDC_RxTx_5ms_sys/69(IRV_u8_TailgateSW_read)  "IRV_u8_TailgateSW"
  run_SWC_FDC_CDD_10ms_sys/11(IRV_u8_TrunkHanSW_write) -> run_SWC_FDC_RxTx_5ms_sys/70(IRV_u8_TrunkHanSW_read)  "IRV_u8_TrunkHanSW"
  run_SWC_FDC_NvmRead_sys/1(IRV_u8Array256_NvmReadArray_write) -> run_SWC_FDC_RxTx_5ms_sys/51(IRV_u8Array256_NvmReadArray_read)  "IRV_u8Array256_NvmReadArray"
  run_SWC_FDC_RxTx_5ms_sys/24(IRV_ms10_CAN1_SG_FD_APS3_write) -> run_SWC_FDC_Tx_10ms_sys/1(IRV_ms10_CAN1_SG_FD_APS3_read)  "IRV_ms10_CAN1_SG_FD_APS3"
  run_SWC_FDC_RxTx_5ms_sys/25(IRV_ms10_CAN1_SG_FD_VCU2_write) -> run_SWC_FDC_Tx_10ms_sys/2(IRV_ms10_CAN1_SG_FD_VCU2_read)  "IRV_ms10_CAN1_SG_FD_VCU2"
  run_SWC_FDC_RxTx_5ms_sys/26(IRV_ms10_CAN1_SG_FD_VCU3_write) -> run_SWC_FDC_Tx_10ms_sys/3(IRV_ms10_CAN1_SG_FD_VCU3_read)  "IRV_ms10_CAN1_SG_FD_VCU3"
  run_SWC_FDC_RxTx_5ms_sys/27(IRV_ms10_CAN2_SG_FD_APS3_write) -> run_SWC_FDC_Tx_10ms_sys/4(IRV_ms10_CAN2_SG_FD_APS3_read)  "IRV_ms10_CAN2_SG_FD_APS3"
  run_SWC_FDC_RxTx_5ms_sys/28(IRV_ms10_CAN2_SG_FD_VCU2_write) -> run_SWC_FDC_Tx_10ms_sys/5(IRV_ms10_CAN2_SG_FD_VCU2_read)  "IRV_ms10_CAN2_SG_FD_VCU2"
  run_SWC_FDC_RxTx_5ms_sys/29(IRV_ms10_CAN3_SG_FD_VCU0_write) -> run_SWC_FDC_Tx_10ms_sys/6(IRV_ms10_CAN3_SG_FD_VCU0_read)  "IRV_ms10_CAN3_SG_FD_VCU0"
  run_SWC_FDC_RxTx_5ms_sys/30(IRV_ms10_CAN3_SG_FD_VCU2_write) -> run_SWC_FDC_Tx_10ms_sys/7(IRV_ms10_CAN3_SG_FD_VCU2_read)  "IRV_ms10_CAN3_SG_FD_VCU2"
  run_SWC_FDC_RxTx_5ms_sys/31(IRV_ms10_CAN5_SG_FD_VCU3_write) -> run_SWC_FDC_Tx_10ms_sys/8(IRV_ms10_CAN5_SG_FD_VCU3_read)  "IRV_ms10_CAN5_SG_FD_VCU3"
  run_SWC_FDC_RxTx_5ms_sys/32(IRV_ms100_CAN1_SG_FD_THCM1_write) -> run_SWC_FDC_Tx_100ms_sys/1(IRV_ms100_CAN1_SG_FD_THCM1_read)  "IRV_ms100_CAN1_SG_FD_THCM1"
  run_SWC_FDC_RxTx_5ms_sys/33(IRV_ms100_CAN2_SG_FD_THCM1_write) -> run_SWC_FDC_Tx_100ms_sys/2(IRV_ms100_CAN2_SG_FD_THCM1_read)  "IRV_ms100_CAN2_SG_FD_THCM1"
  run_SWC_FDC_RxTx_5ms_sys/34(IRV_ms100_CAN3_SG_FD_THCM1_write) -> run_SWC_FDC_Tx_100ms_sys/3(IRV_ms100_CAN3_SG_FD_THCM1_read)  "IRV_ms100_CAN3_SG_FD_THCM1"
  run_SWC_FDC_RxTx_5ms_sys/35(IRV_ms100_CAN4_SG_FD_THCM1_write) -> run_SWC_FDC_Tx_100ms_sys/4(IRV_ms100_CAN4_SG_FD_THCM1_read)  "IRV_ms100_CAN4_SG_FD_THCM1"
  run_SWC_FDC_RxTx_5ms_sys/36(IRV_ms20_CAN1_SG_FD_APS1_write) -> run_SWC_FDC_Tx_20ms_sys/1(IRV_ms20_CAN1_SG_FD_APS1_read)  "IRV_ms20_CAN1_SG_FD_APS1"
  run_SWC_FDC_RxTx_5ms_sys/37(IRV_ms20_CAN1_SG_FD_APS2_write) -> run_SWC_FDC_Tx_20ms_sys/2(IRV_ms20_CAN1_SG_FD_APS2_read)  "IRV_ms20_CAN1_SG_FD_APS2"
  run_SWC_FDC_RxTx_5ms_sys/38(IRV_ms20_CAN2_SG_FD_APS1_write) -> run_SWC_FDC_Tx_20ms_sys/3(IRV_ms20_CAN2_SG_FD_APS1_read)  "IRV_ms20_CAN2_SG_FD_APS1"
  run_SWC_FDC_RxTx_5ms_sys/39(IRV_ms20_CAN2_SG_FD_APS2_write) -> run_SWC_FDC_Tx_20ms_sys/4(IRV_ms20_CAN2_SG_FD_APS2_read)  "IRV_ms20_CAN2_SG_FD_APS2"
  run_SWC_FDC_RxTx_5ms_sys/40(IRV_ms500_CAN2_SG_FD_VCU5_write) -> run_SWC_FDC_Tx_500ms_sys/1(IRV_ms500_CAN2_SG_FD_VCU5_read)  "IRV_ms500_CAN2_SG_FD_VCU5"
  run_SWC_FDC_RxTx_5ms_sys/41(IRV_ms500_CAN5_SG_FD_VCU5_write) -> run_SWC_FDC_Tx_500ms_sys/2(IRV_ms500_CAN5_SG_FD_VCU5_read)  "IRV_ms500_CAN5_SG_FD_VCU5"
  run_SWC_FDC_RxTx_5ms_sys/42(IRV_ms5000_CAN2_SG_FD_VCU6_write) -> run_SWC_FDC_Tx_5000ms_sys/1(IRV_ms5000_CAN2_SG_FD_VCU6_read)  "IRV_ms5000_CAN2_SG_FD_VCU6"
  run_SWC_FDC_RxTx_5ms_sys/43(IRV_E2E_CAN3_SG_FD_VCU1_write) -> run_SWC_FDC_E2E_Write_CAN3VCU1_sys/1(IRV_E2E_CAN3_SG_FD_VCU1_read)  "IRV_E2E_CAN3_SG_FD_VCU1"
  run_SWC_FDC_RxTx_5ms_sys/44(IRV_E2E_CAN4_SG_FD_VCU1_write) -> run_SWC_FDC_E2E_Write_CAN4VCU1_sys/1(IRV_E2E_CAN4_SG_FD_VCU1_read)  "IRV_E2E_CAN4_SG_FD_VCU1"
  run_SWC_FDC_RxTx_5ms_sys/45(IRV_f32_ApsOutVehSpdSig_write) -> run_SWC_FDC_Tx_10ms_sys/9(IRV_f32_ApsOutVehSpdSig_read)  "IRV_f32_ApsOutVehSpdSig"
  run_SWC_FDC_RxTx_5ms_sys/46(IRV_u8Array256_NvmWriteArray_write) -> run_SWC_FDC_NvmWrite_sys/1(IRV_u8Array256_NvmWriteArray_read)  "IRV_u8Array256_NvmWriteArray"
  run_SWC_FDC_RxTx_5ms_sys/47(IRV_u8_ApsOutGearPosnSig_write) -> run_SWC_FDC_Tx_10ms_sys/10(IRV_u8_ApsOutGearPosnSig_read)  "IRV_u8_ApsOutGearPosnSig"
  run_SWC_FDC_RxTx_5ms_sys/48(IRV_u8_ApsOutSendChrgPlugSta_write) -> run_SWC_FDC_Tx_10ms_sys/11(IRV_u8_ApsOutSendChrgPlugSta_read)  "IRV_u8_ApsOutSendChrgPlugSta"
  run_SWC_FDC_RxTx_5ms_sys/49(IRV_u8_ApsOutSetFrSensorOnCmd_write) -> run_SWC_FDC_Tx_10ms_sys/12(IRV_u8_ApsOutSetFrSensorOnCmd_read)  "IRV_u8_ApsOutSetFrSensorOnCmd"
  run_SWC_FDC_RxTx_5ms_sys/50(IRV_u8_ApsOutSetFrSensorSwTOCmd_write) -> run_SWC_FDC_Tx_10ms_sys/13(IRV_u8_ApsOutSetFrSensorSwTOCmd_read)  "IRV_u8_ApsOutSetFrSensorSwTOCmd"
  run_SWC_FDC_RxTx_5ms_sys/51(IRV_u8_ApsOutSetVehSpdTOCmd_write) -> run_SWC_FDC_Tx_10ms_sys/14(IRV_u8_ApsOutSetVehSpdTOCmd_read)  "IRV_u8_ApsOutSetVehSpdTOCmd"
  run_SWC_FDC_Tx_10ms_sys/18(IRV_u8_TPMSDataInSta_write) -> [IRV_u8_TPMSDataInSta_Tag]  "IRV_u8_TPMSDataInSta"
  [IRV_u8_TPMSDataInSta_Tag] -> run_SWC_FDC_RxTx_5ms_sys/68(IRV_u8_TPMSDataInSta_read)
  run_SWC_FDC_Tx_10ms_sys/17(IRV_u8_ApsInSysMode_write) -> [IRV_u8_ApsInSysMode_Tag]  "IRV_u8_ApsInSysMode"
  [IRV_u8_ApsInSysMode_Tag] -> run_SWC_FDC_RxTx_5ms_sys/58(IRV_u8_ApsInSysMode_read)
  run_SWC_FDC_Tx_10ms_sys/16(IRV_u8_ApsInSysFailSta_write) -> [IRV_u8_ApsInSysFailSta_Tag]  "IRV_u8_ApsInSysFailSta"
  [IRV_u8_ApsInSysFailSta_Tag] -> run_SWC_FDC_RxTx_5ms_sys/57(IRV_u8_ApsInSysFailSta_read)
  run_SWC_FDC_Tx_10ms_sys/15(IRV_u8_ApsInSensorLayout_write) -> [IRV_u8_ApsInSensorLayout_Tag]  "IRV_u8_ApsInSensorLayout"
  [IRV_u8_ApsInSensorLayout_Tag] -> run_SWC_FDC_RxTx_5ms_sys/56(IRV_u8_ApsInSensorLayout_read)
  run_SWC_FDC_Tx_10ms_sys/14(IRV_u8_ApsInPASChime_write) -> [IRV_u8_ApsInPASChime_Tag]  "IRV_u8_ApsInPASChime"
  [IRV_u8_ApsInPASChime_Tag] -> run_SWC_FDC_RxTx_5ms_sys/55(IRV_u8_ApsInPASChime_read)
  run_SWC_FDC_Tx_10ms_sys/13(IRV_u8Array9_TPMSData_write) -> [IRV_u8Array9_TPMSData_Tag]  "IRV_u8Array9_TPMSData"
  [IRV_u8Array9_TPMSData_Tag] -> run_SWC_FDC_RxTx_5ms_sys/54(IRV_u8Array9_TPMSData_read)
  run_SWC_FDC_Tx_10ms_sys/12(IRV_u8Array8_PasInDist_write) -> [IRV_u8Array8_PasInDist_Tag]  "IRV_u8Array8_PasInDist"
  [IRV_u8Array8_PasInDist_Tag] -> run_SWC_FDC_RxTx_5ms_sys/53(IRV_u8Array8_PasInDist_read)
  run_SWC_FDC_Tx_10ms_sys/11(IRV_u8Array8_ApsInLevel_write) -> [IRV_u8Array8_ApsInLevel_Tag]  "IRV_u8Array8_ApsInLevel"
  [IRV_u8Array8_ApsInLevel_Tag] -> run_SWC_FDC_RxTx_5ms_sys/52(IRV_u8Array8_ApsInLevel_read)
  run_SWC_FDC_Tx_10ms_sys/10(IRV_u8Array12_ApsInUssSta_write) -> [IRV_u8Array12_ApsInUssSta_Tag]  "IRV_u8Array12_ApsInUssSta"
  [IRV_u8Array12_ApsInUssSta_Tag] -> run_SWC_FDC_RxTx_5ms_sys/50(IRV_u8Array12_ApsInUssSta_read)
  run_SWC_FDC_Tx_10ms_sys/9(IRV_u16Array4_ApsInDist_write) -> [IRV_u16Array4_ApsInDist_Tag]  "IRV_u16Array4_ApsInDist"
  [IRV_u16Array4_ApsInDist_Tag] -> run_SWC_FDC_RxTx_5ms_sys/49(IRV_u16Array4_ApsInDist_read)
  run_SWC_FDC_PAS_1ms/1 -> run_SWC_FDC_PAS_1ms_sys/Trigger
  run_SWC_FDC_UDS_10ms/1 -> run_SWC_FDC_UDS_10ms_sys/Trigger
  run_SWC_FDC_CDD_10ms/1 -> run_SWC_FDC_CDD_10ms_sys/Trigger
  run_SWC_FDC_RxTx_5ms/1 -> run_SWC_FDC_RxTx_5ms_sys/Trigger
  run_SWC_FDC_Tx_10ms/1 -> run_SWC_FDC_Tx_10ms_sys/Trigger
  run_SWC_FDC_Tx_5000ms/1 -> run_SWC_FDC_Tx_5000ms_sys/Trigger
  run_SWC_FDC_Tx_500ms/1 -> run_SWC_FDC_Tx_500ms_sys/Trigger
  run_SWC_FDC_Tx_20ms/1 -> run_SWC_FDC_Tx_20ms_sys/Trigger
  run_SWC_FDC_Tx_100ms/1 -> run_SWC_FDC_Tx_100ms_sys/Trigger

== system SWC_FDC_type/P_WDGCDD ==
  run_SWC_FDC_AppCallWDG_End_sys : Subsystem
  run_SWC_FDC_AppCallWDG_StartUp_sys : Subsystem
  run_SWC_FDC_AppCallWDG_sys : Subsystem

== system SWC_FDC_type/SWC_FDC_type_Init ==
  Event Listener : EventListener  EventName=reset

== system SWC_FDC_type/run_SWC_FDC_AppCallSleep_sys ==
  function : TriggerPort  TriggerType=function-call  IsSimulinkFunction=on  FunctionName=run_SWC_FDC_AppCallSleep  VariantControl=(inherit)
  Constant : Constant  Value=TRUE
  Data Type Conversion : DataTypeConversion  OutDataTypeStr=Enum: AppModeRequestType
  Data Type Conversion1 : DataTypeConversion  OutDataTypeStr=uint8
  P_AppModeReq_requestedMode_write : Outport
  wires:
  Data Type Conversion/1 -> P_AppModeReq_requestedMode_write/1
  Data Type Conversion1/1 -> Data Type Conversion/1
  Constant/1 -> Data Type Conversion1/1

== system SWC_FDC_type/run_SWC_FDC_CDD_10ms_sys ==
  function : TriggerPort  TriggerType=function-call  VariantControl=(inherit)  SampleTimeType=periodic  SampleTime=-1
  R_HALINCDD_CSOP_HALINCDD_IOEXPANDER : FunctionCaller  FunctionPrototype=[u8_HoodSW,u8_TailgateSW,u8_DrDoorSW,u8_PsDoorSW,u8_RRDoorSW,u8_RLDoorSW,u8_CTDSW,u8_HazardSW,u8_TrunkHanSW,u8_SeatSW,u8_CrashSignal] = R_HALINCDD_CSOP_HALINCDD_IOEXPANDER()  OutputArgumentSpecifications=uint8(1), uint8(1), uint8(1), uint8(1), uint8(1), uint8(1), uint8(1), uint8(1), uint8(1), uint8(1), uint8(1)
  IRV_u8_CTDSW_write : Outport  OutDataTypeStr=uint8  PortDimensions=1
  IRV_u8_CrashSignal_write : Outport  Port=2  OutDataTypeStr=uint8  PortDimensions=1
  IRV_u8_DrDoorSW_write : Outport  Port=3  OutDataTypeStr=uint8  PortDimensions=1
  IRV_u8_HazardSW_write : Outport  Port=4  OutDataTypeStr=uint8  PortDimensions=1
  IRV_u8_HoodSW_write : Outport  Port=5  OutDataTypeStr=uint8  PortDimensions=1
  IRV_u8_PsDoorSW_write : Outport  Port=6  OutDataTypeStr=uint8  PortDimensions=1
  IRV_u8_RLDoorSW_write : Outport  Port=7  OutDataTypeStr=uint8  PortDimensions=1
  IRV_u8_RRDoorSW_write : Outport  Port=8  OutDataTypeStr=uint8  PortDimensions=1
  IRV_u8_SeatSW_write : Outport  Port=9  OutDataTypeStr=uint8  PortDimensions=1
  IRV_u8_TailgateSW_write : Outport  Port=10  OutDataTypeStr=uint8  PortDimensions=1
  IRV_u8_TrunkHanSW_write : Outport  Port=11  OutDataTypeStr=uint8  PortDimensions=1
  wires:
  R_HALINCDD_CSOP_HALINCDD_IOEXPANDER/1 -> IRV_u8_HoodSW_write/1
  R_HALINCDD_CSOP_HALINCDD_IOEXPANDER/2 -> IRV_u8_TailgateSW_write/1
  R_HALINCDD_CSOP_HALINCDD_IOEXPANDER/3 -> IRV_u8_DrDoorSW_write/1
  R_HALINCDD_CSOP_HALINCDD_IOEXPANDER/4 -> IRV_u8_PsDoorSW_write/1
  R_HALINCDD_CSOP_HALINCDD_IOEXPANDER/5 -> IRV_u8_RRDoorSW_write/1
  R_HALINCDD_CSOP_HALINCDD_IOEXPANDER/6 -> IRV_u8_RLDoorSW_write/1
  R_HALINCDD_CSOP_HALINCDD_IOEXPANDER/7 -> IRV_u8_CTDSW_write/1
  R_HALINCDD_CSOP_HALINCDD_IOEXPANDER/8 -> IRV_u8_HazardSW_write/1
  R_HALINCDD_CSOP_HALINCDD_IOEXPANDER/9 -> IRV_u8_TrunkHanSW_write/1
  R_HALINCDD_CSOP_HALINCDD_IOEXPANDER/10 -> IRV_u8_SeatSW_write/1
  R_HALINCDD_CSOP_HALINCDD_IOEXPANDER/11 -> IRV_u8_CrashSignal_write/1

== system SWC_FDC_type/run_SWC_FDC_E2E_Write_CAN3VCU1_sys ==
  IRV_E2E_CAN3_SG_FD_VCU1_read : Inport
  function : TriggerPort  TriggerType=function-call  IsSimulinkFunction=on  FunctionName=run_SWC_FDC_E2E_Write_CAN3VCU1  VariantControl=(inherit)
  P_CAN3_FD_VCU1_CAN3_SG_FD_VCU1_write : Outport
  wires:
  IRV_E2E_CAN3_SG_FD_VCU1_read/1 -> P_CAN3_FD_VCU1_CAN3_SG_FD_VCU1_write/1

== system SWC_FDC_type/run_SWC_FDC_E2E_Write_CAN4VCU1_sys ==
  IRV_E2E_CAN4_SG_FD_VCU1_read : Inport
  function : TriggerPort  TriggerType=function-call  IsSimulinkFunction=on  FunctionName=run_SWC_FDC_E2E_Write_CAN4VCU1  VariantControl=(inherit)
  P_CAN4_FD_VCU1_CAN4_SG_FD_VCU1_write : Outport
  wires:
  IRV_E2E_CAN4_SG_FD_VCU1_read/1 -> P_CAN4_FD_VCU1_CAN4_SG_FD_VCU1_write/1

== system SWC_FDC_type/run_SWC_FDC_NvmRead_sys ==
  R_NVMRead_NV_FVTDataArray_read : Inport
  function : TriggerPort  TriggerType=function-call  IsSimulinkFunction=on  FunctionName=run_SWC_FDC_NvmRead  VariantControl=(inherit)
  IRV_u8Array256_NvmReadArray_write : Outport  OutDataTypeStr=uint8  PortDimensions=256
  wires:
  R_NVMRead_NV_FVTDataArray_read/1 -> IRV_u8Array256_NvmReadArray_write/1

== system SWC_FDC_type/run_SWC_FDC_NvmWrite_sys ==
  IRV_u8Array256_NvmWriteArray_read : Inport
  function : TriggerPort  TriggerType=function-call  IsSimulinkFunction=on  FunctionName=run_SWC_FDC_NvmWrite  VariantControl=(inherit)
  P_NVMWrite_NV_FVTDataArray_write : Outport
  wires:
  IRV_u8Array256_NvmWriteArray_read/1 -> P_NVMWrite_NV_FVTDataArray_write/1

== system SWC_FDC_type/run_SWC_FDC_PAS_1ms_sys ==
  function : TriggerPort  TriggerType=function-call  VariantControl=(inherit)  SampleTimeType=periodic  SampleTime=-1
  R_HALINCDD_CSOP_PAS_Handler : FunctionCaller  FunctionPrototype=R_HALINCDD_CSOP_PAS_Handler()
